simulink model "latesttopology"  (Simulink 8.4)
settings: Solver=ode23tb  StartTime=0.0  StopTime=1  MaxStep=0.0001  MinStep=0.00001  RelTol=1e-3
undefined symbols (not defined in the file): sigbuilder_block
libraries: powerlib x88, simulink x10, powerlib_meascontrol x1
settings Model: Creator=SELVA  LastModifiedBy=SELVA
settings ConfigurationSet: Description=SimMechanics 2G

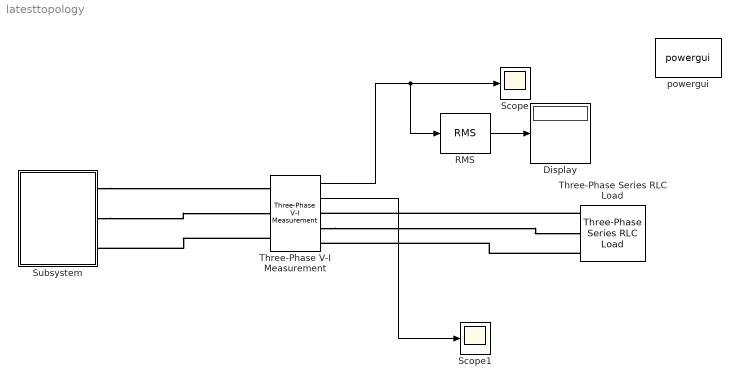
== system latesttopology ==
  Display : Display
  RMS : powerlib_meascontrol/Measurements/RMS  TrueRMS=on  Freq=50  RMSInit=0  Ts=0
  Scope : Scope
      settings: YMin=-800  YMax=800
  Scope1 : Scope
      settings: YMin=-800  YMax=800
  Subsystem : Subsystem  mask{v=65, fc=1000, m=1}
      mask prompts: v "DC Voltage"; fc "Switching Frequency"; m "Modulation Index"
  Three-Phase Series RLC Load : powerlib/Elements/Three-Phase Series RLC Load  LConnTagsString=A|B|C  Configuration=Y (grounded)  NominalVoltage=410  NominalFrequency=50  ActivePower=1e3  InductivePower=00  CapacitivePower=00  Measurements=None  LoadType=constant Z
  Three-Phase V-I Measurement : powerlib/Measurements/Three-Phase V-I Measurement  VoltageMeasurement=phase-to-phase  SetLabelV=off  LabelV=Vabc  Vpu=off  VpuLL=off  CurrentMeasurement=yes  SetLabelI=off  LabelI=Iabc  Ipu=off  Pbase=100e6  Vbase=500e3  OutputType=Complex  PhasorSimulation=off  PSBequivalent=0
  powergui : powerlib/powergui  Priority=1  SimulationMode=Discrete  SolverType=Tustin/Backward Euler (TBE)  SampleTime=50e-6  frequency=60  SPID=off  DisableSnubberDevices=off  DisableRonSwitches=off  DisableVfSwitches=off  SwTol=0  DisplayEquations=off  Interpol=off  methode=off  Ts=100  frequencyindice=0  Pbase=100e6  ErrMax=1e-4  Iterations=50  UnitsV=kV  UnitsW=MW  FunctionMessages=off  echomessages=off  HookPort=off  EnableUseOfTLC=off  x0status=blocks  RestoreLinks=warning  ResistiveCurrentMeasurement=off  Frange=[0:2:500]  Ylog=off  Xlog=on  ShowGrid=off  save=off  variable=ZData  structure=0  ZoomFFT=off  StartTime=0.0  cycles=1  DisplayStyle=1  fundamental=60  FreqAxis=off  MaxFrequency=1000  frequencyindicesteady=1  RmsSteady=1  display=off
  wires:
  Three-Phase V-I Measurement/1 -> RMS/1, Scope/1
  RMS/1 -> Display/1
  Three-Phase V-I Measurement/2 -> Scope1/1
  connections:
  Subsystem/RConn1 -- Three-Phase V-I Measurement/LConn1
  Subsystem/RConn2 -- Three-Phase V-I Measurement/LConn2
  Three-Phase V-I Measurement/LConn3 -- Subsystem/RConn3
  Three-Phase Series RLC Load/LConn1 -- Three-Phase V-I Measurement/RConn1
  Three-Phase V-I Measurement/RConn2 -- Three-Phase Series RLC Load/LConn2
  Three-Phase Series RLC Load/LConn3 -- Three-Phase V-I Measurement/RConn3

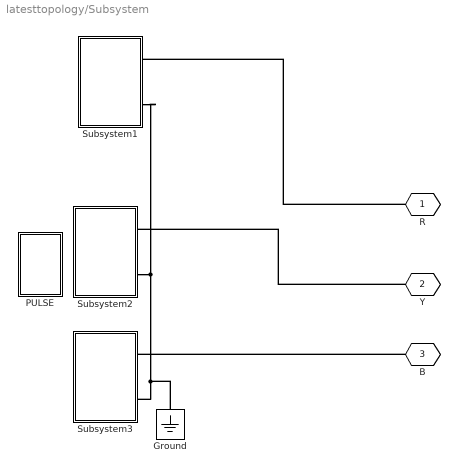
== system latesttopology/Subsystem ==
  Ground : powerlib/Elements/Ground  LConnTagsString=a
  PULSE : Subsystem
  Subsystem1 : Subsystem
  Subsystem2 : Subsystem
  Subsystem3 : Subsystem
  R : PMIOPort  Port=1  Side=Right
  Y : PMIOPort  Port=2  Side=Right
  B : PMIOPort  Port=3  Side=Right
  connections:
  Subsystem1/RConn2 -- Subsystem2/RConn2 -- Ground/LConn1 -- Subsystem3/RConn2
  B/RConn1 -- Subsystem3/RConn1
  R/RConn1 -- Subsystem1/RConn1
  Y/RConn1 -- Subsystem2/RConn1

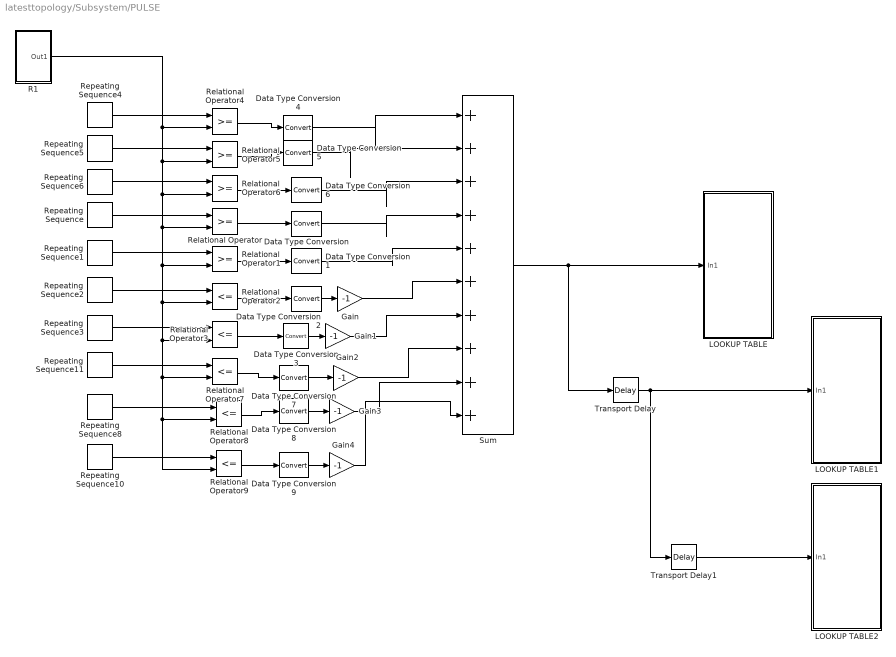
== system latesttopology/Subsystem/PULSE ==
  Data Type Conversion{,1..9} (10 alike) : DataTypeConversion
  Gain{,1..4} (5 alike) : Gain  Gain=-1
  LOOKUP TABLE : Subsystem
  LOOKUP TABLE1 : Subsystem
  LOOKUP TABLE2 : Subsystem
  R1 : Subsystem
  Relational Operator{,1,4..6} (5 alike) : RelationalOperator  OutDataTypeStr=boolean
  Relational Operator{2..3,7..9} (5 alike) : RelationalOperator  Operator=<=  OutDataTypeStr=boolean
  Repeating Sequence : simulink/Sources/Repeating Sequence  rep_seq_t="[0 (1/fc)/2  (1/fc)]"  rep_seq_y=[2 1 2]
  Repeating Sequence1 : simulink/Sources/Repeating Sequence  rep_seq_t="[0 (1/fc)/2  (1/fc)]"  rep_seq_y=[1 0 1]
  Repeating Sequence10 : simulink/Sources/Repeating Sequence  rep_seq_t="[0 (1/fc)/2  (1/fc)]"  rep_seq_y=[-5 -4 -5]
  Repeating Sequence11 : simulink/Sources/Repeating Sequence  rep_seq_t="[0 (1/fc)/2  (1/fc)]"  rep_seq_y=[-3 -2 -3]
  Repeating Sequence2 : simulink/Sources/Repeating Sequence  rep_seq_t="[0 (1/fc)/2  (1/fc)]"  rep_seq_y=[-1 0 -1]
  Repeating Sequence3 : simulink/Sources/Repeating Sequence  rep_seq_t="[0 (1/fc)/2  (1/fc)]"  rep_seq_y=[-2 -1 -2]
  Repeating Sequence4 : simulink/Sources/Repeating Sequence  rep_seq_t="[0 (1/fc)/2  (1/fc)]"  rep_seq_y=[4 5 4]
  Repeating Sequence5 : simulink/Sources/Repeating Sequence  rep_seq_t="[0 (1/fc)/2  (1/fc)]"  rep_seq_y=[4 3 4]
  Repeating Sequence6 : simulink/Sources/Repeating Sequence  rep_seq_t="[0 (1/fc)/2  (1/fc)]"  rep_seq_y=[3 2 3]
  Repeating Sequence8 : simulink/Sources/Repeating Sequence  rep_seq_t="[0 (1/fc)/2  (1/fc)]"  rep_seq_y=[-4 -3 -4]
  Sum : Sum  Inputs=|++++++++++
  Transport Delay : TransportDelay  DelayTime=(2/3)*0.01
  Transport Delay1 : TransportDelay  DelayTime=(2/3)*0.01
  wires:
  Data Type Conversion3/1 -> Gain1/1
  Data Type Conversion2/1 -> Gain/1
  Relational Operator3/1 -> Data Type Conversion3/1
  Relational Operator2/1 -> Data Type Conversion2/1
  Repeating Sequence3/1 -> Relational Operator3/1
  Repeating Sequence2/1 -> Relational Operator2/1
  Repeating Sequence1/1 -> Relational Operator1/1
  Repeating Sequence/1 -> Relational Operator/1
  Relational Operator1/1 -> Data Type Conversion1/1
  Relational Operator/1 -> Data Type Conversion/1
  Repeating Sequence6/1 -> Relational Operator6/1
  Repeating Sequence5/1 -> Relational Operator5/1
  Repeating Sequence4/1 -> Relational Operator4/1
  Relational Operator6/1 -> Data Type Conversion6/1
  Relational Operator5/1 -> Data Type Conversion5/1
  Relational Operator4/1 -> Data Type Conversion4/1
  Repeating Sequence8/1 -> Relational Operator8/1
  Repeating Sequence11/1 -> Relational Operator7/1
  Relational Operator9/1 -> Data Type Conversion9/1
  Relational Operator8/1 -> Data Type Conversion8/1
  Relational Operator7/1 -> Data Type Conversion7/1
  Data Type Conversion9/1 -> Gain4/1
  Data Type Conversion8/1 -> Gain3/1
  Data Type Conversion7/1 -> Gain2/1
  Repeating Sequence10/1 -> Relational Operator9/1
  Data Type Conversion4/1 -> Sum/1
  Data Type Conversion5/1 -> Sum/2
  Data Type Conversion6/1 -> Sum/3
  Data Type Conversion/1 -> Sum/4
  Data Type Conversion1/1 -> Sum/5
  Gain/1 -> Sum/6
  Gain1/1 -> Sum/7
  Gain2/1 -> Sum/8
  Gain3/1 -> Sum/9
  Gain4/1 -> Sum/10
  R1/1(Out1) -> Relational Operator4/2, Relational Operator5/2, Relational Operator6/2, Relational Operator1/2, Relational Operator2/2, Relational Operator3/2, Relational Operator7/2, Relational Operator8/2, Relational Operator9/2, Relational Operator/2
  Sum/1 -> Transport Delay/1, LOOKUP TABLE/1(In1)
  Transport Delay/1 -> LOOKUP TABLE1/1(In1), Transport Delay1/1
  Transport Delay1/1 -> LOOKUP TABLE2/1(In1)

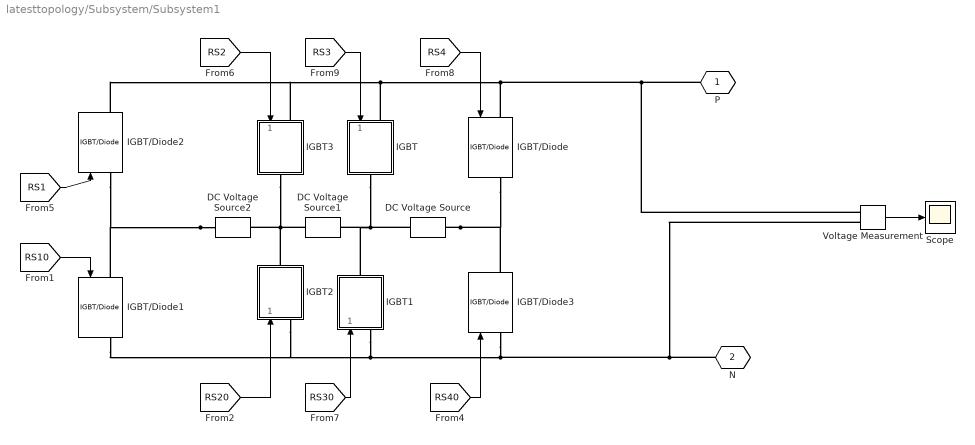
== system latesttopology/Subsystem/Subsystem1 ==
  DC Voltage Source : powerlib/Electrical Sources/DC Voltage Source  Amplitude=v  Measurements=None
  DC Voltage Source1 : powerlib/Electrical Sources/DC Voltage Source  Amplitude=2*v  Measurements=None
  DC Voltage Source2 : powerlib/Electrical Sources/DC Voltage Source  Amplitude=2*v  Measurements=None
  IGBT : Subsystem
  IGBT/Diode{,1..3} (4 alike) : powerlib/Power Electronics/IGBT//Diode  Ron=1e-3  Rs=1e5  Cs=inf  Measurements=on
  IGBT1 : Subsystem
  IGBT2 : Subsystem
  IGBT3 : Subsystem
  Scope : Scope
      settings: YMin=-50  YMax=50  SaveName=ScopeData2
  Voltage Measurement : powerlib/Measurements/Voltage Measurement  PhasorSimulation=off  OutputType=Complex  PSBequivalent=0
  P : PMIOPort  Port=1  Side=Right
  N : PMIOPort  Port=2  Side=Right
  wires:
  Voltage Measurement/1 -> Scope/1
  [RS1] -> IGBT/Diode2/1
  [RS4] -> IGBT/Diode/1
  [RS10] -> IGBT/Diode1/1
  [RS40] -> IGBT/Diode3/1
  [RS2] -> IGBT3/1(Gate)
  [RS3] -> IGBT/1(Gate)
  [RS20] -> IGBT2/1(Gate)
  [RS30] -> IGBT1/1(Gate)
  connections:
  DC Voltage Source1/RConn1 -- IGBT3/RConn1 -- IGBT2/RConn1 -- DC Voltage Source2/LConn1
  DC Voltage Source/RConn1 -- IGBT1/RConn1 -- DC Voltage Source1/LConn1 -- IGBT/RConn1
  Voltage Measurement/LConn1 -- P/RConn1 -- IGBT/Diode/LConn1 -- IGBT/Diode2/RConn1 -- IGBT3/LConn1 -- IGBT/LConn1
  Voltage Measurement/LConn2 -- N/RConn1 -- IGBT/Diode3/LConn1 -- IGBT1/LConn1 -- IGBT/Diode1/RConn1 -- IGBT2/LConn1
  DC Voltage Source/LConn1 -- IGBT/Diode3/RConn1 -- IGBT/Diode/RConn1
  DC Voltage Source2/RConn1 -- IGBT/Diode1/LConn1 -- IGBT/Diode2/LConn1

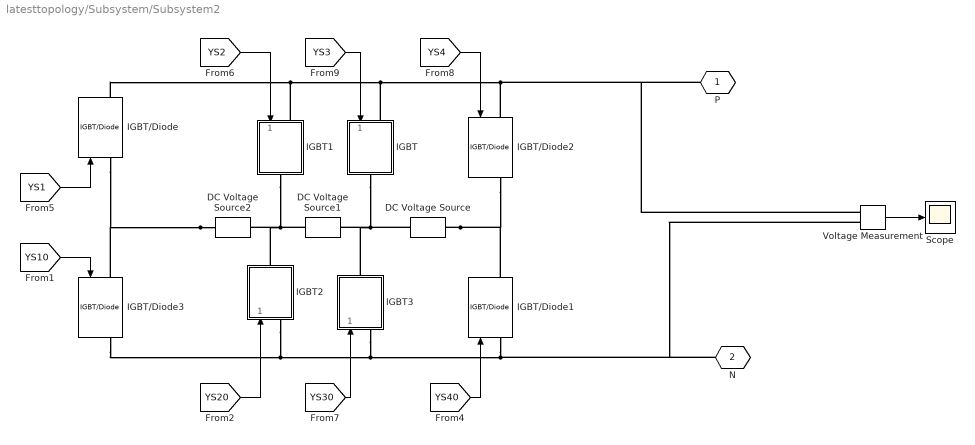
== system latesttopology/Subsystem/Subsystem2 ==
  DC Voltage Source : powerlib/Electrical Sources/DC Voltage Source  Amplitude=v  Measurements=None
  DC Voltage Source1 : powerlib/Electrical Sources/DC Voltage Source  Amplitude=2*v  Measurements=None
  DC Voltage Source2 : powerlib/Electrical Sources/DC Voltage Source  Amplitude=2*v  Measurements=None
  IGBT : Subsystem
  IGBT/Diode{,1..3} (4 alike) : powerlib/Power Electronics/IGBT//Diode  Ron=1e-3  Rs=1e5  Cs=inf  Measurements=on
  IGBT1 : Subsystem
  IGBT2 : Subsystem
  IGBT3 : Subsystem
  Scope : Scope
      settings: YMin=-50  YMax=50  SaveName=ScopeData2
  Voltage Measurement : powerlib/Measurements/Voltage Measurement  PhasorSimulation=off  OutputType=Complex  PSBequivalent=0
  P : PMIOPort  Port=1  Side=Right
  N : PMIOPort  Port=2  Side=Right
  wires:
  [YS30] -> IGBT3/1(Gate)
  [YS20] -> IGBT2/1(Gate)
  [YS3] -> IGBT/1(Gate)
  [YS2] -> IGBT1/1(Gate)
  [YS40] -> IGBT/Diode1/1
  [YS10] -> IGBT/Diode3/1
  [YS4] -> IGBT/Diode2/1
  [YS1] -> IGBT/Diode/1
  Voltage Measurement/1 -> Scope/1
  connections:
  DC Voltage Source2/RConn1 -- IGBT/Diode3/LConn1 -- IGBT/Diode/LConn1
  DC Voltage Source/LConn1 -- IGBT/Diode2/RConn1 -- IGBT/Diode1/RConn1
  IGBT/Diode3/RConn1 -- IGBT2/LConn1 -- IGBT3/LConn1 -- IGBT/Diode1/LConn1 -- N/RConn1 -- Voltage Measurement/LConn2
  IGBT/Diode/RConn1 -- IGBT1/LConn1 -- IGBT/LConn1 -- IGBT/Diode2/LConn1 -- P/RConn1 -- Voltage Measurement/LConn1
  DC Voltage Source/RConn1 -- IGBT3/RConn1 -- DC Voltage Source1/LConn1 -- IGBT/RConn1
  DC Voltage Source1/RConn1 -- IGBT2/RConn1 -- DC Voltage Source2/LConn1 -- IGBT1/RConn1

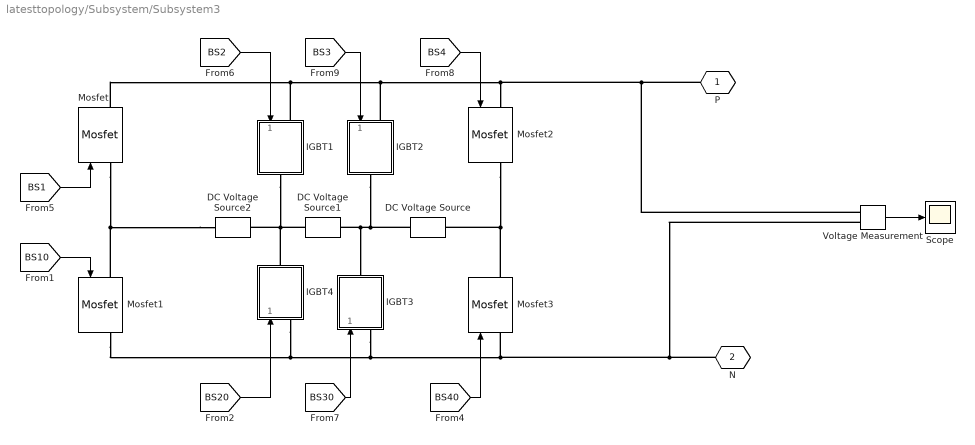
== system latesttopology/Subsystem/Subsystem3 ==
  DC Voltage Source : powerlib/Electrical Sources/DC Voltage Source  Amplitude=v  Measurements=None
  DC Voltage Source1 : powerlib/Electrical Sources/DC Voltage Source  Amplitude=2*v  Measurements=None
  DC Voltage Source2 : powerlib/Electrical Sources/DC Voltage Source  Amplitude=2*v  Measurements=None
  IGBT1 : Subsystem
  IGBT2 : Subsystem
  IGBT3 : Subsystem
  IGBT4 : Subsystem
  Mosfet{,1..3} (4 alike) : powerlib/Power Electronics/Mosfet  Ron=0.1  Lon=0  Rd=0.01  Vfd=0  IC=0  Rs=1e5  Cs=inf  Measurements=on
  Scope : Scope
      settings: YMin=-50  YMax=50  SaveName=ScopeData2
  Voltage Measurement : powerlib/Measurements/Voltage Measurement  PhasorSimulation=off  OutputType=Complex  PSBequivalent=0
  P : PMIOPort  Port=1  Side=Right
  N : PMIOPort  Port=2  Side=Right
  wires:
  Voltage Measurement/1 -> Scope/1
  [BS1] -> Mosfet/1
  [BS4] -> Mosfet2/1
  [BS10] -> Mosfet1/1
  [BS40] -> Mosfet3/1
  [BS2] -> IGBT1/1(Gate)
  [BS3] -> IGBT2/1(Gate)
  [BS20] -> IGBT4/1(Gate)
  [BS30] -> IGBT3/1(Gate)
  connections:
  DC Voltage Source2/LConn1 -- IGBT4/RConn1 -- IGBT1/RConn1 -- DC Voltage Source1/RConn1
  DC Voltage Source1/LConn1 -- IGBT2/RConn1 -- DC Voltage Source/RConn1 -- IGBT3/RConn1
  Mosfet/RConn1 -- IGBT1/LConn1 -- IGBT2/LConn1 -- Voltage Measurement/LConn1 -- P/RConn1 -- Mosfet2/LConn1
  IGBT3/LConn1 -- Mosfet1/RConn1 -- IGBT4/LConn1 -- Voltage Measurement/LConn2 -- N/RConn1 -- Mosfet3/LConn1
  Mosfet3/RConn1 -- Mosfet2/RConn1 -- DC Voltage Source/LConn1
  DC Voltage Source2/RConn1 -- Mosfet/LConn1 -- Mosfet1/LConn1

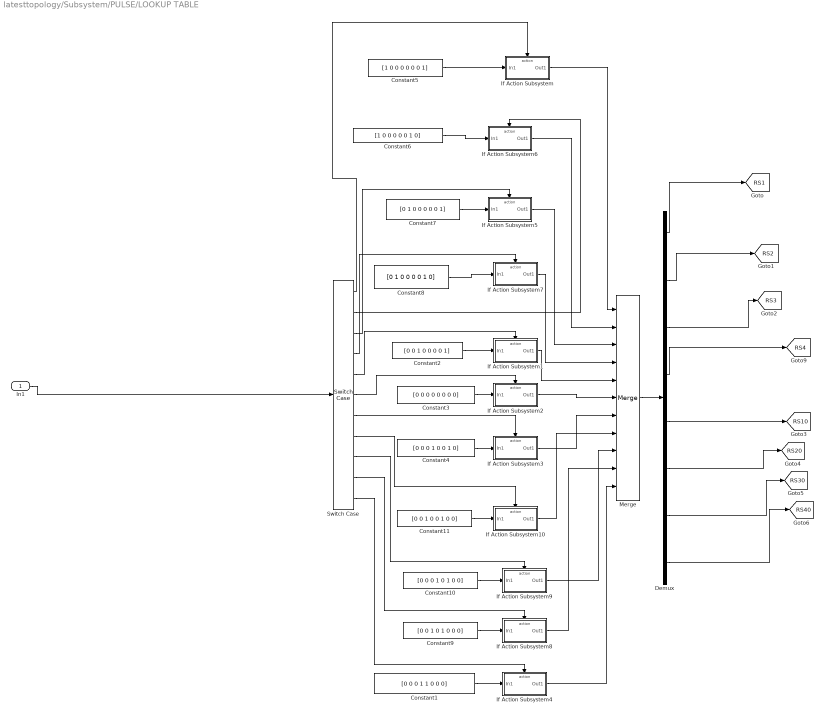
== system latesttopology/Subsystem/PULSE/LOOKUP TABLE ==
  In1 : Inport
  Constant1 : Constant  Value=[0 0 0 1 1 0 0 0]
  Constant10 : Constant  Value=[0 0 0 1 0 1 0 0]
  Constant11 : Constant  Value=[0 0 1 0 0 1 0 0]
  Constant2 : Constant  Value=[0 0 1 0 0 0 0 1]
  Constant3 : Constant  Value=[0 0 0 0 0 0 0 0]
  Constant4 : Constant  Value=[0 0 0 1 0 0 1 0]
  Constant5 : Constant  Value=[1 0 0 0 0 0 0 1]
  Constant6 : Constant  Value=[1 0 0 0 0 0 1 0]
  Constant7 : Constant  Value=[0 1 0 0 0 0 0 1]
  Constant8 : Constant  Value=[0 1 0 0 0 0 1 0]
  Constant9 : Constant  Value=[0 0 1 0 1 0 0 0]
  Demux : Demux  Outputs=8
  If Action Subsystem : Subsystem  TreatAsAtomicUnit=on
  If Action Subsystem1 : Subsystem  TreatAsAtomicUnit=on
  If Action Subsystem10 : Subsystem  TreatAsAtomicUnit=on
  If Action Subsystem2 : Subsystem  TreatAsAtomicUnit=on
  If Action Subsystem3 : Subsystem  TreatAsAtomicUnit=on
  If Action Subsystem4 : Subsystem  TreatAsAtomicUnit=on
  If Action Subsystem5 : Subsystem  TreatAsAtomicUnit=on
  If Action Subsystem6 : Subsystem  TreatAsAtomicUnit=on
  If Action Subsystem7 : Subsystem  TreatAsAtomicUnit=on
  If Action Subsystem8 : Subsystem  TreatAsAtomicUnit=on
  If Action Subsystem9 : Subsystem  TreatAsAtomicUnit=on
  Merge : Merge  Inputs=11
  Switch Case : SwitchCase  CaseConditions={-5 -4 -3 -2 -1 0 1 2 3 4 5}  ShowDefaultCase=off
  tag scope: RS10=global, RS1=global, RS20=global, RS2=global, RS30=global, RS3=global, RS40=global, RS4=global
  wires:
  Merge/1 -> Demux/1
  If Action Subsystem/1(Out1) -> Merge/1
  Constant4/1 -> If Action Subsystem3/1(In1)
  Constant3/1 -> If Action Subsystem2/1(In1)
  Constant2/1 -> If Action Subsystem1/1(In1)
  Switch Case/6 -> If Action Subsystem2/Action
  If Action Subsystem6/1(Out1) -> Merge/2
  If Action Subsystem5/1(Out1) -> Merge/3
  If Action Subsystem7/1(Out1) -> Merge/4
  If Action Subsystem1/1(Out1) -> Merge/5
  If Action Subsystem2/1(Out1) -> Merge/6
  If Action Subsystem3/1(Out1) -> Merge/7
  Constant9/1 -> If Action Subsystem8/1(In1)
  Constant10/1 -> If Action Subsystem9/1(In1)
  Constant11/1 -> If Action Subsystem10/1(In1)
  Switch Case/11 -> If Action Subsystem4/Action
  If Action Subsystem4/1(Out1) -> Merge/11
  Switch Case/10 -> If Action Subsystem8/Action
  Switch Case/9 -> If Action Subsystem9/Action
  Switch Case/8 -> If Action Subsystem10/Action
  Switch Case/7 -> If Action Subsystem3/Action
  Switch Case/5 -> If Action Subsystem1/Action
  Switch Case/4 -> If Action Subsystem7/Action
  Switch Case/3 -> If Action Subsystem5/Action
  Switch Case/2 -> If Action Subsystem6/Action
  Switch Case/1 -> If Action Subsystem/Action
  Constant6/1 -> If Action Subsystem6/1(In1)
  Constant7/1 -> If Action Subsystem5/1(In1)
  Constant8/1 -> If Action Subsystem7/1(In1)
  If Action Subsystem10/1(Out1) -> Merge/8
  If Action Subsystem9/1(Out1) -> Merge/9
  If Action Subsystem8/1(Out1) -> Merge/10
  Demux/3 -> [RS3]
  Demux/2 -> [RS2]
  Demux/1 -> [RS1]
  Demux/4 -> [RS4]
  Constant1/1 -> If Action Subsystem4/1(In1)
  Constant5/1 -> If Action Subsystem/1(In1)
  In1/1 -> Switch Case/1
  Demux/5 -> [RS10]
  Demux/6 -> [RS20]
  Demux/7 -> [RS30]
  Demux/8 -> [RS40]

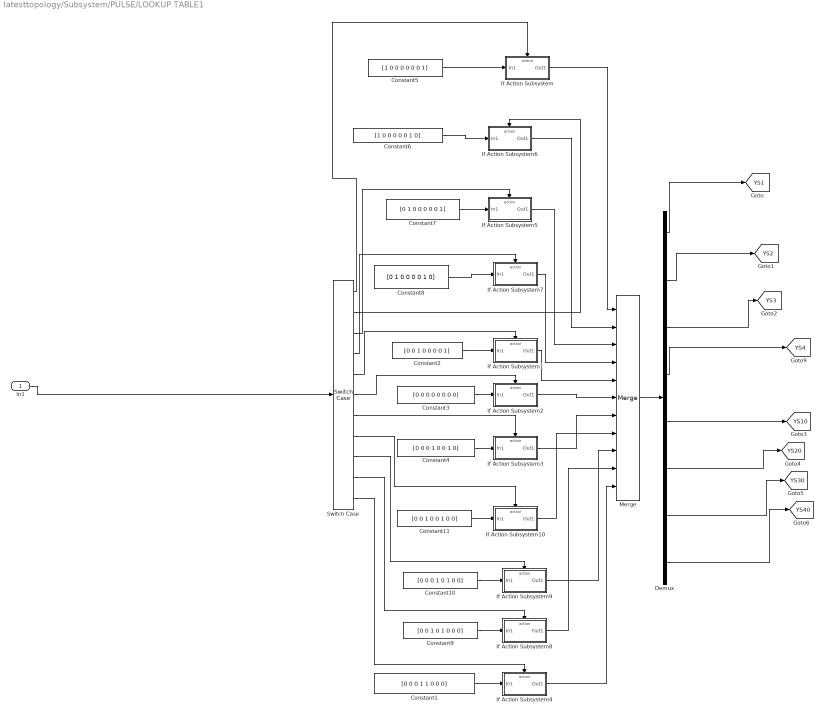
== system latesttopology/Subsystem/PULSE/LOOKUP TABLE1 ==
  In1 : Inport
  Constant1 : Constant  Value=[0 0 0 1 1 0 0 0]
  Constant10 : Constant  Value=[0 0 0 1 0 1 0 0]
  Constant11 : Constant  Value=[0 0 1 0 0 1 0 0]
  Constant2 : Constant  Value=[0 0 1 0 0 0 0 1]
  Constant3 : Constant  Value=[0 0 0 0 0 0 0 0]
  Constant4 : Constant  Value=[0 0 0 1 0 0 1 0]
  Constant5 : Constant  Value=[1 0 0 0 0 0 0 1]
  Constant6 : Constant  Value=[1 0 0 0 0 0 1 0]
  Constant7 : Constant  Value=[0 1 0 0 0 0 0 1]
  Constant8 : Constant  Value=[0 1 0 0 0 0 1 0]
  Constant9 : Constant  Value=[0 0 1 0 1 0 0 0]
  Demux : Demux  Outputs=8
  If Action Subsystem : Subsystem  TreatAsAtomicUnit=on
  If Action Subsystem1 : Subsystem  TreatAsAtomicUnit=on
  If Action Subsystem10 : Subsystem  TreatAsAtomicUnit=on
  If Action Subsystem2 : Subsystem  TreatAsAtomicUnit=on
  If Action Subsystem3 : Subsystem  TreatAsAtomicUnit=on
  If Action Subsystem4 : Subsystem  TreatAsAtomicUnit=on
  If Action Subsystem5 : Subsystem  TreatAsAtomicUnit=on
  If Action Subsystem6 : Subsystem  TreatAsAtomicUnit=on
  If Action Subsystem7 : Subsystem  TreatAsAtomicUnit=on
  If Action Subsystem8 : Subsystem  TreatAsAtomicUnit=on
  If Action Subsystem9 : Subsystem  TreatAsAtomicUnit=on
  Merge : Merge  Inputs=11
  Switch Case : SwitchCase  CaseConditions={-5 -4 -3 -2 -1 0 1 2 3 4 5}  ShowDefaultCase=off
  tag scope: YS10=global, YS1=global, YS20=global, YS2=global, YS30=global, YS3=global, YS40=global, YS4=global
  wires:
  Demux/8 -> [YS40]
  Demux/7 -> [YS30]
  Demux/6 -> [YS20]
  Demux/5 -> [YS10]
  In1/1 -> Switch Case/1
  Constant5/1 -> If Action Subsystem/1(In1)
  Constant1/1 -> If Action Subsystem4/1(In1)
  Demux/4 -> [YS4]
  Demux/1 -> [YS1]
  Demux/2 -> [YS2]
  Demux/3 -> [YS3]
  If Action Subsystem8/1(Out1) -> Merge/10
  If Action Subsystem9/1(Out1) -> Merge/9
  If Action Subsystem10/1(Out1) -> Merge/8
  Constant8/1 -> If Action Subsystem7/1(In1)
  Constant7/1 -> If Action Subsystem5/1(In1)
  Constant6/1 -> If Action Subsystem6/1(In1)
  Switch Case/1 -> If Action Subsystem/Action
  Switch Case/2 -> If Action Subsystem6/Action
  Switch Case/3 -> If Action Subsystem5/Action
  Switch Case/4 -> If Action Subsystem7/Action
  Switch Case/5 -> If Action Subsystem1/Action
  Switch Case/7 -> If Action Subsystem3/Action
  Switch Case/8 -> If Action Subsystem10/Action
  Switch Case/9 -> If Action Subsystem9/Action
  Switch Case/10 -> If Action Subsystem8/Action
  If Action Subsystem4/1(Out1) -> Merge/11
  Switch Case/11 -> If Action Subsystem4/Action
  Constant11/1 -> If Action Subsystem10/1(In1)
  Constant10/1 -> If Action Subsystem9/1(In1)
  Constant9/1 -> If Action Subsystem8/1(In1)
  If Action Subsystem3/1(Out1) -> Merge/7
  If Action Subsystem2/1(Out1) -> Merge/6
  If Action Subsystem1/1(Out1) -> Merge/5
  If Action Subsystem7/1(Out1) -> Merge/4
  If Action Subsystem5/1(Out1) -> Merge/3
  If Action Subsystem6/1(Out1) -> Merge/2
  Switch Case/6 -> If Action Subsystem2/Action
  Constant2/1 -> If Action Subsystem1/1(In1)
  Constant3/1 -> If Action Subsystem2/1(In1)
  Constant4/1 -> If Action Subsystem3/1(In1)
  If Action Subsystem/1(Out1) -> Merge/1
  Merge/1 -> Demux/1

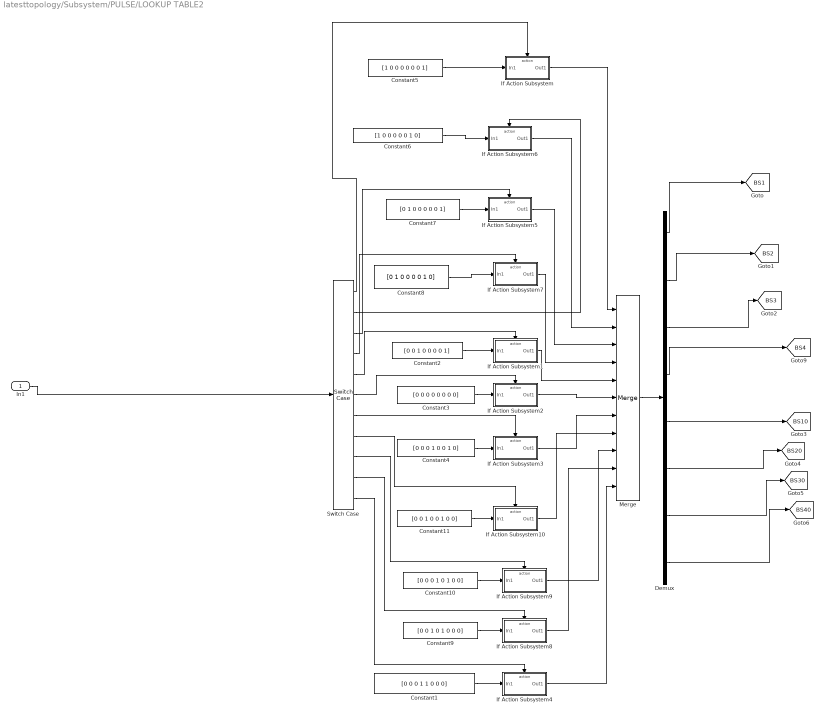
== system latesttopology/Subsystem/PULSE/LOOKUP TABLE2 ==
  In1 : Inport
  Constant1 : Constant  Value=[0 0 0 1 1 0 0 0]
  Constant10 : Constant  Value=[0 0 0 1 0 1 0 0]
  Constant11 : Constant  Value=[0 0 1 0 0 1 0 0]
  Constant2 : Constant  Value=[0 0 1 0 0 0 0 1]
  Constant3 : Constant  Value=[0 0 0 0 0 0 0 0]
  Constant4 : Constant  Value=[0 0 0 1 0 0 1 0]
  Constant5 : Constant  Value=[1 0 0 0 0 0 0 1]
  Constant6 : Constant  Value=[1 0 0 0 0 0 1 0]
  Constant7 : Constant  Value=[0 1 0 0 0 0 0 1]
  Constant8 : Constant  Value=[0 1 0 0 0 0 1 0]
  Constant9 : Constant  Value=[0 0 1 0 1 0 0 0]
  Demux : Demux  Outputs=8
  If Action Subsystem : Subsystem  TreatAsAtomicUnit=on
  If Action Subsystem1 : Subsystem  TreatAsAtomicUnit=on
  If Action Subsystem10 : Subsystem  TreatAsAtomicUnit=on
  If Action Subsystem2 : Subsystem  TreatAsAtomicUnit=on
  If Action Subsystem3 : Subsystem  TreatAsAtomicUnit=on
  If Action Subsystem4 : Subsystem  TreatAsAtomicUnit=on
  If Action Subsystem5 : Subsystem  TreatAsAtomicUnit=on
  If Action Subsystem6 : Subsystem  TreatAsAtomicUnit=on
  If Action Subsystem7 : Subsystem  TreatAsAtomicUnit=on
  If Action Subsystem8 : Subsystem  TreatAsAtomicUnit=on
  If Action Subsystem9 : Subsystem  TreatAsAtomicUnit=on
  Merge : Merge  Inputs=11
  Switch Case : SwitchCase  CaseConditions={-5 -4 -3 -2 -1 0 1 2 3 4 5}  ShowDefaultCase=off
  tag scope: BS10=global, BS1=global, BS20=global, BS2=global, BS30=global, BS3=global, BS40=global, BS4=global
  wires:
  Merge/1 -> Demux/1
  If Action Subsystem/1(Out1) -> Merge/1
  Constant4/1 -> If Action Subsystem3/1(In1)
  Constant3/1 -> If Action Subsystem2/1(In1)
  Constant2/1 -> If Action Subsystem1/1(In1)
  Switch Case/6 -> If Action Subsystem2/Action
  If Action Subsystem6/1(Out1) -> Merge/2
  If Action Subsystem5/1(Out1) -> Merge/3
  If Action Subsystem7/1(Out1) -> Merge/4
  If Action Subsystem1/1(Out1) -> Merge/5
  If Action Subsystem2/1(Out1) -> Merge/6
  If Action Subsystem3/1(Out1) -> Merge/7
  Constant9/1 -> If Action Subsystem8/1(In1)
  Constant10/1 -> If Action Subsystem9/1(In1)
  Constant11/1 -> If Action Subsystem10/1(In1)
  Switch Case/11 -> If Action Subsystem4/Action
  If Action Subsystem4/1(Out1) -> Merge/11
  Switch Case/10 -> If Action Subsystem8/Action
  Switch Case/9 -> If Action Subsystem9/Action
  Switch Case/8 -> If Action Subsystem10/Action
  Switch Case/7 -> If Action Subsystem3/Action
  Switch Case/5 -> If Action Subsystem1/Action
  Switch Case/4 -> If Action Subsystem7/Action
  Switch Case/3 -> If Action Subsystem5/Action
  Switch Case/2 -> If Action Subsystem6/Action
  Switch Case/1 -> If Action Subsystem/Action
  Constant6/1 -> If Action Subsystem6/1(In1)
  Constant7/1 -> If Action Subsystem5/1(In1)
  Constant8/1 -> If Action Subsystem7/1(In1)
  If Action Subsystem10/1(Out1) -> Merge/8
  If Action Subsystem9/1(Out1) -> Merge/9
  If Action Subsystem8/1(Out1) -> Merge/10
  Demux/3 -> [BS3]
  Demux/2 -> [BS2]
  Demux/1 -> [BS1]
  Demux/4 -> [BS4]
  Constant1/1 -> If Action Subsystem4/1(In1)
  Constant5/1 -> If Action Subsystem/1(In1)
  In1/1 -> Switch Case/1
  Demux/5 -> [BS10]
  Demux/6 -> [BS20]
  Demux/7 -> [BS30]
  Demux/8 -> [BS40]

== system latesttopology/Subsystem/PULSE/R1 ==
  Product : Product
  Signal Builder : Subsystem  Tag=STV Subsys  LoadFcn=sigbuilder_block('load');  StartFcn=sigbuilder_block('start');  StopFcn=sigbuilder_block('stop');  ClipboardFcn=sigbuilder_block('clipboard');  mask(Sigbuilder block){}
      mask help: Simulink:masks:SigbuilderBlock_MD
      mask init:
      | if ~strcmp(get_param(bdroot(gcbh),'SimulationStatus'),'stopped') tuvar = sigbuilder_block('maskInit'); end
      settings: CopyFcn=sigbuilder_block('copy');  DeleteFcn=sigbuilder_block('delete');  ModelCloseFcn=sigbuilder_block('modelClose');  PreSaveFcn=sigbuilder_block('preSave');  PauseFcn=sigbuilder_block('pause');  ContinueFcn=sigbuilder_block('continue');  NameChangeFcn=sigbuilder_block('namechange');  OpenFcn=sigbuilder_block('open',[437.6 199.2 550.4 400 ]);  CloseFcn=sigbuilder_block('close');
      mask Display: plot(0, 0, 100, 100,[2, 2, 32, 32, 2], [68, 8, 8, 68, 68],[32, 2], [38, 38], [32, 19, 2],[53, 60, 44], [32, 17, 17, 2],[16, 16, 31, 31]);txt = getActiveGroup(gcbh);text(2, 100, txt,'verticalAlignment', 'top');
  Sine Wave : Sin  Amplitude=5*m  Frequency=2*pi*50  SampleTime=0
  Out1 : Outport
  wires:
  Sine Wave/1 -> Out1/1, Product/1
  Signal Builder/1(Signal 1) -> Product/2

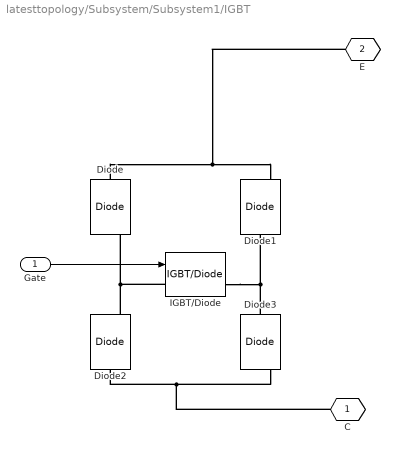
== system latesttopology/Subsystem/Subsystem1/IGBT ==
  Gate : Inport
  Diode{,1..3} (4 alike) : powerlib/Power Electronics/Diode  Ron=0.001  Lon=0  Vf=0.8  IC=0  UseSnubber=off  Rs=500  Cs=250e-9  Measurements=on
  IGBT/Diode : powerlib/Power Electronics/IGBT//Diode  Ron=1e-3  Rs=1e5  Cs=inf  Measurements=on
  C : PMIOPort  Port=1  Side=Left
  E : PMIOPort  Port=2  Side=Right
  wires:
  Gate/1 -> IGBT/Diode/1
  connections:
  Diode2/RConn1 -- IGBT/Diode/LConn1 -- Diode/RConn1
  Diode3/LConn1 -- IGBT/Diode/RConn1 -- Diode1/LConn1
  Diode3/RConn1 -- C/RConn1 -- Diode2/LConn1
  Diode/LConn1 -- E/RConn1 -- Diode1/RConn1

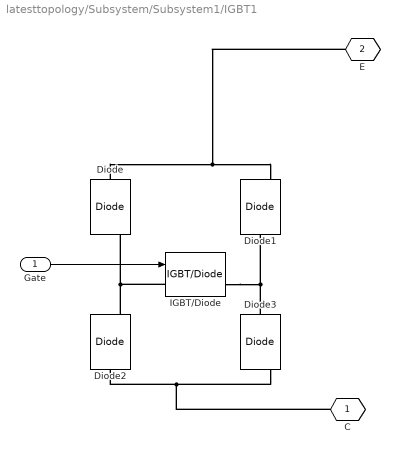
== system latesttopology/Subsystem/Subsystem1/IGBT1 ==
  Gate : Inport
  Diode{,1..3} (4 alike) : powerlib/Power Electronics/Diode  Ron=0.001  Lon=0  Vf=0.8  IC=0  UseSnubber=off  Rs=500  Cs=250e-9  Measurements=on
  IGBT/Diode : powerlib/Power Electronics/IGBT//Diode  Ron=1e-3  Rs=1e5  Cs=inf  Measurements=on
  C : PMIOPort  Port=1  Side=Left
  E : PMIOPort  Port=2  Side=Right
  wires:
  Gate/1 -> IGBT/Diode/1
  connections:
  E/RConn1 -- Diode/LConn1 -- Diode1/RConn1
  C/RConn1 -- Diode3/RConn1 -- Diode2/LConn1
  IGBT/Diode/RConn1 -- Diode3/LConn1 -- Diode1/LConn1
  IGBT/Diode/LConn1 -- Diode2/RConn1 -- Diode/RConn1

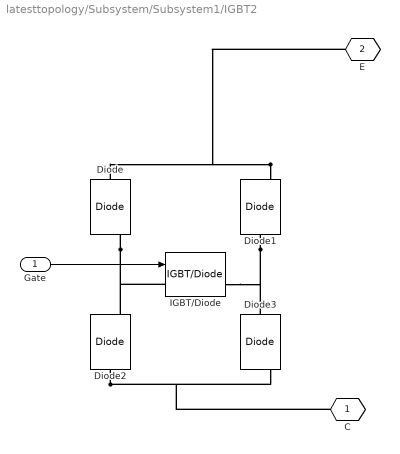
== system latesttopology/Subsystem/Subsystem1/IGBT2 ==
  Gate : Inport
  Diode{,1..3} (4 alike) : powerlib/Power Electronics/Diode  Ron=0.001  Lon=0  Vf=0.8  IC=0  UseSnubber=off  Rs=500  Cs=250e-9  Measurements=on
  IGBT/Diode : powerlib/Power Electronics/IGBT//Diode  Ron=1e-3  Rs=1e5  Cs=inf  Measurements=on
  C : PMIOPort  Port=1  Side=Left
  E : PMIOPort  Port=2  Side=Right
  wires:
  Gate/1 -> IGBT/Diode/1
  connections:
  Diode/RConn1 -- Diode2/RConn1 -- IGBT/Diode/LConn1
  Diode1/LConn1 -- Diode3/LConn1 -- IGBT/Diode/RConn1
  Diode2/LConn1 -- Diode3/RConn1 -- C/RConn1
  Diode1/RConn1 -- Diode/LConn1 -- E/RConn1

== system latesttopology/Subsystem/Subsystem1/IGBT3 ==
  Gate : Inport
  Diode{,1..3} (4 alike) : powerlib/Power Electronics/Diode  Ron=0.001  Lon=0  Vf=0.8  IC=0  UseSnubber=off  Rs=500  Cs=250e-9  Measurements=on
  IGBT/Diode : powerlib/Power Electronics/IGBT//Diode  Ron=1e-3  Rs=1e5  Cs=inf  Measurements=on
  C : PMIOPort  Port=1  Side=Left
  E : PMIOPort  Port=2  Side=Right
  wires:
  Gate/1 -> IGBT/Diode/1
  connections:
  E/RConn1 -- Diode/LConn1 -- Diode1/RConn1
  C/RConn1 -- Diode3/RConn1 -- Diode2/LConn1
  IGBT/Diode/RConn1 -- Diode3/LConn1 -- Diode1/LConn1
  IGBT/Diode/LConn1 -- Diode2/RConn1 -- Diode/RConn1

== system latesttopology/Subsystem/Subsystem2/IGBT ==
  Gate : Inport
  Diode{,1..3} (4 alike) : powerlib/Power Electronics/Diode  Ron=0.001  Lon=0  Vf=0.8  IC=0  UseSnubber=off  Rs=500  Cs=250e-9  Measurements=on
  IGBT/Diode : powerlib/Power Electronics/IGBT//Diode  Ron=1e-3  Rs=1e5  Cs=inf  Measurements=on
  C : PMIOPort  Port=1  Side=Left
  E : PMIOPort  Port=2  Side=Right
  wires:
  Gate/1 -> IGBT/Diode/1
  connections:
  Diode/RConn1 -- Diode2/RConn1 -- IGBT/Diode/LConn1
  Diode1/LConn1 -- Diode3/LConn1 -- IGBT/Diode/RConn1
  Diode2/LConn1 -- Diode3/RConn1 -- C/RConn1
  Diode1/RConn1 -- Diode/LConn1 -- E/RConn1

== system latesttopology/Subsystem/Subsystem2/IGBT1 ==
  Gate : Inport
  Diode{,1..3} (4 alike) : powerlib/Power Electronics/Diode  Ron=0.001  Lon=0  Vf=0.8  IC=0  UseSnubber=off  Rs=500  Cs=250e-9  Measurements=on
  IGBT/Diode : powerlib/Power Electronics/IGBT//Diode  Ron=1e-3  Rs=1e5  Cs=inf  Measurements=on
  C : PMIOPort  Port=1  Side=Left
  E : PMIOPort  Port=2  Side=Right
  wires:
  Gate/1 -> IGBT/Diode/1
  connections:
  E/RConn1 -- Diode/LConn1 -- Diode1/RConn1
  C/RConn1 -- Diode3/RConn1 -- Diode2/LConn1
  IGBT/Diode/RConn1 -- Diode3/LConn1 -- Diode1/LConn1
  IGBT/Diode/LConn1 -- Diode2/RConn1 -- Diode/RConn1

== system latesttopology/Subsystem/Subsystem2/IGBT2 ==
  Gate : Inport
  Diode{,1..3} (4 alike) : powerlib/Power Electronics/Diode  Ron=0.001  Lon=0  Vf=0.8  IC=0  UseSnubber=off  Rs=500  Cs=250e-9  Measurements=on
  IGBT/Diode : powerlib/Power Electronics/IGBT//Diode  Ron=1e-3  Rs=1e5  Cs=inf  Measurements=on
  C : PMIOPort  Port=1  Side=Left
  E : PMIOPort  Port=2  Side=Right
  wires:
  Gate/1 -> IGBT/Diode/1
  connections:
  Diode/RConn1 -- Diode2/RConn1 -- IGBT/Diode/LConn1
  Diode1/LConn1 -- Diode3/LConn1 -- IGBT/Diode/RConn1
  Diode2/LConn1 -- Diode3/RConn1 -- C/RConn1
  Diode1/RConn1 -- Diode/LConn1 -- E/RConn1

== system latesttopology/Subsystem/Subsystem2/IGBT3 ==
  Gate : Inport
  Diode{,1..3} (4 alike) : powerlib/Power Electronics/Diode  Ron=0.001  Lon=0  Vf=0.8  IC=0  UseSnubber=off  Rs=500  Cs=250e-9  Measurements=on
  IGBT/Diode : powerlib/Power Electronics/IGBT//Diode  Ron=1e-3  Rs=1e5  Cs=inf  Measurements=on
  C : PMIOPort  Port=1  Side=Left
  E : PMIOPort  Port=2  Side=Right
  wires:
  Gate/1 -> IGBT/Diode/1
  connections:
  E/RConn1 -- Diode/LConn1 -- Diode1/RConn1
  C/RConn1 -- Diode3/RConn1 -- Diode2/LConn1
  IGBT/Diode/RConn1 -- Diode3/LConn1 -- Diode1/LConn1
  IGBT/Diode/LConn1 -- Diode2/RConn1 -- Diode/RConn1

== system latesttopology/Subsystem/Subsystem3/IGBT1 ==
  Gate : Inport
  Diode{,1..3} (4 alike) : powerlib/Power Electronics/Diode  Ron=0.001  Lon=0  Vf=0.8  IC=0  UseSnubber=off  Rs=500  Cs=250e-9  Measurements=on
  IGBT/Diode : powerlib/Power Electronics/IGBT//Diode  Ron=1e-3  Rs=1e5  Cs=inf  Measurements=on
  C : PMIOPort  Port=1  Side=Left
  E : PMIOPort  Port=2  Side=Right
  wires:
  Gate/1 -> IGBT/Diode/1
  connections:
  E/RConn1 -- Diode/LConn1 -- Diode1/RConn1
  C/RConn1 -- Diode3/RConn1 -- Diode2/LConn1
  IGBT/Diode/RConn1 -- Diode3/LConn1 -- Diode1/LConn1
  IGBT/Diode/LConn1 -- Diode2/RConn1 -- Diode/RConn1

== system latesttopology/Subsystem/Subsystem3/IGBT2 ==
  Gate : Inport
  Diode{,1..3} (4 alike) : powerlib/Power Electronics/Diode  Ron=0.001  Lon=0  Vf=0.8  IC=0  UseSnubber=off  Rs=500  Cs=250e-9  Measurements=on
  IGBT/Diode : powerlib/Power Electronics/IGBT//Diode  Ron=1e-3  Rs=1e5  Cs=inf  Measurements=on
  C : PMIOPort  Port=1  Side=Left
  E : PMIOPort  Port=2  Side=Right
  wires:
  Gate/1 -> IGBT/Diode/1
  connections:
  Diode/RConn1 -- Diode2/RConn1 -- IGBT/Diode/LConn1
  Diode1/LConn1 -- Diode3/LConn1 -- IGBT/Diode/RConn1
  Diode2/LConn1 -- Diode3/RConn1 -- C/RConn1
  Diode1/RConn1 -- Diode/LConn1 -- E/RConn1

== system latesttopology/Subsystem/Subsystem3/IGBT3 ==
  Gate : Inport
  Diode{,1..3} (4 alike) : powerlib/Power Electronics/Diode  Ron=0.001  Lon=0  Vf=0.8  IC=0  UseSnubber=off  Rs=500  Cs=250e-9  Measurements=on
  IGBT/Diode : powerlib/Power Electronics/IGBT//Diode  Ron=1e-3  Rs=1e5  Cs=inf  Measurements=on
  C : PMIOPort  Port=1  Side=Left
  E : PMIOPort  Port=2  Side=Right
  wires:
  Gate/1 -> IGBT/Diode/1
  connections:
  E/RConn1 -- Diode/LConn1 -- Diode1/RConn1
  C/RConn1 -- Diode3/RConn1 -- Diode2/LConn1
  IGBT/Diode/RConn1 -- Diode3/LConn1 -- Diode1/LConn1
  IGBT/Diode/LConn1 -- Diode2/RConn1 -- Diode/RConn1

== system latesttopology/Subsystem/Subsystem3/IGBT4 ==
  Gate : Inport
  Diode{,1..3} (4 alike) : powerlib/Power Electronics/Diode  Ron=0.001  Lon=0  Vf=0.8  IC=0  UseSnubber=off  Rs=500  Cs=250e-9  Measurements=on
  IGBT/Diode : powerlib/Power Electronics/IGBT//Diode  Ron=1e-3  Rs=1e5  Cs=inf  Measurements=on
  C : PMIOPort  Port=1  Side=Left
  E : PMIOPort  Port=2  Side=Right
  wires:
  Gate/1 -> IGBT/Diode/1
  connections:
  Diode/RConn1 -- Diode2/RConn1 -- IGBT/Diode/LConn1
  Diode1/LConn1 -- Diode3/LConn1 -- IGBT/Diode/RConn1
  Diode2/LConn1 -- Diode3/RConn1 -- C/RConn1
  Diode1/RConn1 -- Diode/LConn1 -- E/RConn1

== system latesttopology/Subsystem/PULSE/LOOKUP TABLE/If Action Subsystem ==
  In1 : Inport
  Action Port : ActionPort  ActionType=case
  Out1 : Outport
  wires:
  In1/1 -> Out1/1

== system latesttopology/Subsystem/PULSE/LOOKUP TABLE/If Action Subsystem1 ==
  In1 : Inport
  Action Port : ActionPort  ActionType=case
  Out1 : Outport
  wires:
  In1/1 -> Out1/1

== system latesttopology/Subsystem/PULSE/LOOKUP TABLE/If Action Subsystem10 ==
  In1 : Inport
  Action Port : ActionPort  ActionType=case
  Out1 : Outport
  wires:
  In1/1 -> Out1/1

== system latesttopology/Subsystem/PULSE/LOOKUP TABLE/If Action Subsystem2 ==
  In1 : Inport
  Action Port : ActionPort  ActionType=case
  Out1 : Outport
  wires:
  In1/1 -> Out1/1

== system latesttopology/Subsystem/PULSE/LOOKUP TABLE/If Action Subsystem3 ==
  In1 : Inport
  Action Port : ActionPort  ActionType=case
  Out1 : Outport
  wires:
  In1/1 -> Out1/1

== system latesttopology/Subsystem/PULSE/LOOKUP TABLE/If Action Subsystem4 ==
  In1 : Inport
  Action Port : ActionPort  ActionType=case
  Out1 : Outport
  wires:
  In1/1 -> Out1/1

== system latesttopology/Subsystem/PULSE/LOOKUP TABLE/If Action Subsystem5 ==
  In1 : Inport
  Action Port : ActionPort  ActionType=case
  Out1 : Outport
  wires:
  In1/1 -> Out1/1

== system latesttopology/Subsystem/PULSE/LOOKUP TABLE/If Action Subsystem6 ==
  In1 : Inport
  Action Port : ActionPort  ActionType=case
  Out1 : Outport
  wires:
  In1/1 -> Out1/1

== system latesttopology/Subsystem/PULSE/LOOKUP TABLE/If Action Subsystem7 ==
  In1 : Inport
  Action Port : ActionPort  ActionType=case
  Out1 : Outport
  wires:
  In1/1 -> Out1/1

== system latesttopology/Subsystem/PULSE/LOOKUP TABLE/If Action Subsystem8 ==
  In1 : Inport
  Action Port : ActionPort  ActionType=case
  Out1 : Outport
  wires:
  In1/1 -> Out1/1

== system latesttopology/Subsystem/PULSE/LOOKUP TABLE/If Action Subsystem9 ==
  In1 : Inport
  Action Port : ActionPort  ActionType=case
  Out1 : Outport
  wires:
  In1/1 -> Out1/1

== system latesttopology/Subsystem/PULSE/LOOKUP TABLE1/If Action Subsystem ==
  In1 : Inport
  Action Port : ActionPort  ActionType=case
  Out1 : Outport
  wires:
  In1/1 -> Out1/1

== system latesttopology/Subsystem/PULSE/LOOKUP TABLE1/If Action Subsystem1 ==
  In1 : Inport
  Action Port : ActionPort  ActionType=case
  Out1 : Outport
  wires:
  In1/1 -> Out1/1

== system latesttopology/Subsystem/PULSE/LOOKUP TABLE1/If Action Subsystem10 ==
  In1 : Inport
  Action Port : ActionPort  ActionType=case
  Out1 : Outport
  wires:
  In1/1 -> Out1/1

== system latesttopology/Subsystem/PULSE/LOOKUP TABLE1/If Action Subsystem2 ==
  In1 : Inport
  Action Port : ActionPort  ActionType=case
  Out1 : Outport
  wires:
  In1/1 -> Out1/1

== system latesttopology/Subsystem/PULSE/LOOKUP TABLE1/If Action Subsystem3 ==
  In1 : Inport
  Action Port : ActionPort  ActionType=case
  Out1 : Outport
  wires:
  In1/1 -> Out1/1

== system latesttopology/Subsystem/PULSE/LOOKUP TABLE1/If Action Subsystem4 ==
  In1 : Inport
  Action Port : ActionPort  ActionType=case
  Out1 : Outport
  wires:
  In1/1 -> Out1/1

== system latesttopology/Subsystem/PULSE/LOOKUP TABLE1/If Action Subsystem5 ==
  In1 : Inport
  Action Port : ActionPort  ActionType=case
  Out1 : Outport
  wires:
  In1/1 -> Out1/1

== system latesttopology/Subsystem/PULSE/LOOKUP TABLE1/If Action Subsystem6 ==
  In1 : Inport
  Action Port : ActionPort  ActionType=case
  Out1 : Outport
  wires:
  In1/1 -> Out1/1

== system latesttopology/Subsystem/PULSE/LOOKUP TABLE1/If Action Subsystem7 ==
  In1 : Inport
  Action Port : ActionPort  ActionType=case
  Out1 : Outport
  wires:
  In1/1 -> Out1/1

== system latesttopology/Subsystem/PULSE/LOOKUP TABLE1/If Action Subsystem8 ==
  In1 : Inport
  Action Port : ActionPort  ActionType=case
  Out1 : Outport
  wires:
  In1/1 -> Out1/1

== system latesttopology/Subsystem/PULSE/LOOKUP TABLE1/If Action Subsystem9 ==
  In1 : Inport
  Action Port : ActionPort  ActionType=case
  Out1 : Outport
  wires:
  In1/1 -> Out1/1

== system latesttopology/Subsystem/PULSE/LOOKUP TABLE2/If Action Subsystem ==
  In1 : Inport
  Action Port : ActionPort  ActionType=case
  Out1 : Outport
  wires:
  In1/1 -> Out1/1

== system latesttopology/Subsystem/PULSE/LOOKUP TABLE2/If Action Subsystem1 ==
  In1 : Inport
  Action Port : ActionPort  ActionType=case
  Out1 : Outport
  wires:
  In1/1 -> Out1/1

== system latesttopology/Subsystem/PULSE/LOOKUP TABLE2/If Action Subsystem10 ==
  In1 : Inport
  Action Port : ActionPort  ActionType=case
  Out1 : Outport
  wires:
  In1/1 -> Out1/1

== system latesttopology/Subsystem/PULSE/LOOKUP TABLE2/If Action Subsystem2 ==
  In1 : Inport
  Action Port : ActionPort  ActionType=case
  Out1 : Outport
  wires:
  In1/1 -> Out1/1

== system latesttopology/Subsystem/PULSE/LOOKUP TABLE2/If Action Subsystem3 ==
  In1 : Inport
  Action Port : ActionPort  ActionType=case
  Out1 : Outport
  wires:
  In1/1 -> Out1/1

== system latesttopology/Subsystem/PULSE/LOOKUP TABLE2/If Action Subsystem4 ==
  In1 : Inport
  Action Port : ActionPort  ActionType=case
  Out1 : Outport
  wires:
  In1/1 -> Out1/1

== system latesttopology/Subsystem/PULSE/LOOKUP TABLE2/If Action Subsystem5 ==
  In1 : Inport
  Action Port : ActionPort  ActionType=case
  Out1 : Outport
  wires:
  In1/1 -> Out1/1

== system latesttopology/Subsystem/PULSE/LOOKUP TABLE2/If Action Subsystem6 ==
  In1 : Inport
  Action Port : ActionPort  ActionType=case
  Out1 : Outport
  wires:
  In1/1 -> Out1/1

== system latesttopology/Subsystem/PULSE/LOOKUP TABLE2/If Action Subsystem7 ==
  In1 : Inport
  Action Port : ActionPort  ActionType=case
  Out1 : Outport
  wires:
  In1/1 -> Out1/1

== system latesttopology/Subsystem/PULSE/LOOKUP TABLE2/If Action Subsystem8 ==
  In1 : Inport
  Action Port : ActionPort  ActionType=case
  Out1 : Outport
  wires:
  In1/1 -> Out1/1

== system latesttopology/Subsystem/PULSE/LOOKUP TABLE2/If Action Subsystem9 ==
  In1 : Inport
  Action Port : ActionPort  ActionType=case
  Out1 : Outport
  wires:
  In1/1 -> Out1/1

== system latesttopology/Subsystem/PULSE/R1/Signal Builder ==
  Demux : Demux  Tag=STV Demux  Outputs=1
  FromWs : FromWorkspace  Tag=STV FromWs  VariableName=tuvar  SampleTime=0  SigBuilderData=DataTag0  VnvData=DataTag1
      SigBuilderData=|
      | common.afterFinalStr = 'Extrapolate'
      | common.sampleTime = 0
      | dataSet.timeRange = [0 5]
      | dataSet.name = 'Group 1'
      | sbobj.Groups.Name = 'Group 1'
      | sbobj.Groups.Signals.Name = 'Signal 1'
      | sbobj.Groups.Signals.XData = [0 0.1 0.2 0.304 0.44 0.44 3 3 5]
      | sbobj.Groups.Signals.YData = [0.505 0.505 0.505 0.505 0.505 0.605 0.605 1 1]
      | sbobj.Groups.TimeRange = [0 5]
  Signal 1 : Outport  Tag=STV Outport
  wires:
  Demux/1 -> Signal 1/1
  FromWs/1 -> Demux/1
